simulink model "vending_machine_model"  (R2020a)
settings: Solver=FixedStepAuto  StartTime=0.0  StopTime=20.0  FixedStep=1  RelTol=1e-3
settings Model: Creator=Viraj  LastModifiedBy=Viraj

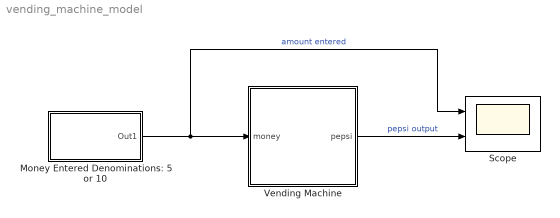
== system vending_machine_model ==
  Money Entered Denominations: 5 or 10 : Subsystem
      mask Display: image('Capture.JPG'); % Use "Edit Image" on toolstrip to change.
  Scope : Scope  NumInputPorts=2
  Vending Machine : Stateflow chart  TreatAsAtomicUnit=on
  wires:
  Money Entered Denominations: 5 or 10/1(Out1) -> Scope/1, Vending Machine/1(money)  "amount entered"
  Vending Machine/1(pepsi) -> Scope/2  "pepsi output"

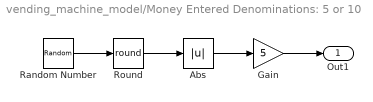
== system vending_machine_model/Money Entered Denominations: 5 or 10 ==
  Abs : Abs
  Gain : Gain  Gain=5
  Random Number : RandomNumber  SampleTime=1
  Round : Rounding  Operator=round
  Out1 : Outport
  wires:
  Gain/1 -> Out1/1
  Random Number/1 -> Round/1
  Round/1 -> Abs/1
  Abs/1 -> Gain/1

== stateflow chart vending_machine_model/Vending Machine ==
  state zero_in_machine
  state five_in_machine
  state ten_in_machine
  (default) -> zero_in_machine
  zero_in_machine -> five_in_machine [order 1] : [money == 5]{pepsi = 0}
  five_in_machine -> zero_in_machine [order 2] : [money == 10]{pepsi = 1}
  ten_in_machine -> zero_in_machine [order 1] : [money == 5]{pepsi = 1}
  zero_in_machine -> ten_in_machine [order 2] : [money == 10]{pepsi = 0}
  five_in_machine -> ten_in_machine [order 1] : [money == 5]{pepsi = 0}
  ten_in_machine -> five_in_machine [order 2] : [money == 10]{pepsi = 1}
  data: money input; pepsi output
